simulink model "LAB4"  (R2023b)
settings: Solver=FixedStepDiscrete  StartTime=0.0  StopTime=Inf  FixedStep=0.02  RelTol=1e-3  EnableMultiTasking=on
model workspace (MAT data in the model file):
  SL_ROS_VariableLengthArrays_MaxSizes : object (value not decoded)
values from neighbouring files (symbols this model uses):
  x = x + offset    [lab4.m]    (also in occupancy_map.m; occupancy_map2.m)
  x_path = x_path(4:4:end)    [lab4.m]
  y = y + offset    [lab4.m]    (also in occupancy_map.m; occupancy_map2.m)
  y_path = y_path(4:4:end)    [lab4.m]
undefined symbols (not defined in the file or in its folder): angdiff, Angular, Linear
libraries: simulink x5, robotlib x4, robotcorelib x1, simulink_extras x1
(part 2 of 2)

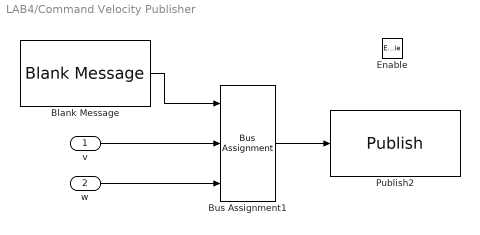
== system LAB4/Command Velocity Publisher ==
  v : Inport
  w : Inport  Port=2
  Enable : EnablePort
  Blank Message : robotlib/Blank Message  messageClass=Message  entityType=geometry_msgs/Twist  messageType=geometry_msgs/Twist  SampleTime=inf  legacyBusStruct=off
  Bus Assignment1 : BusAssignment  DialogController=Simulink.DDGSource_BusAssignment  AssignedSignals=Linear.X,Angular.Z
  Publish2 : robotlib/Publish  topicSource=Select from ROS network  topic=/cmd_vel  messageType=geometry_msgs/Twist  legacyBusStruct=off  messageQueueLength=105
  wires:
  Bus Assignment1/1 -> Publish2/1
  Blank Message/1 -> Bus Assignment1/1
  v/1 -> Bus Assignment1/2
  w/1 -> Bus Assignment1/3

== system LAB4/More Info ==

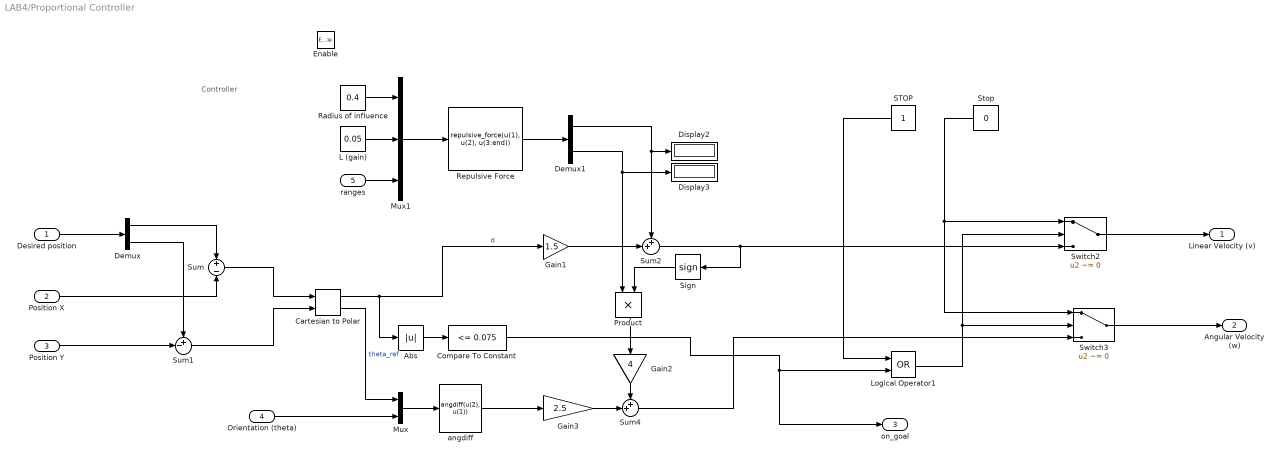
== system LAB4/Proportional Controller ==
  note: Controller
  Desired position : Inport
  Position X : Inport  Port=2
  Position Y : Inport  Port=3
  Orientation (theta) : Inport  Port=4
  ranges : Inport  Port=5
  Enable : EnablePort
  Abs : Abs  SaturateOnIntegerOverflow=off
  Cartesian to Polar : simulink_extras/Transformations/Cartesian to Polar
  Compare To Constant : simulink/Logic and Bit Operations/Compare To Constant  relop=<=  const=0.075  OutDataTypeStr=boolean
  Demux : Demux  Outputs=2
  Demux1 : Demux  Outputs=2
  Display2 : Display
  Display3 : Display
  Gain1 : Gain  Gain=1.5
  Gain2 : Gain  Gain=4
  Gain3 : Gain  Gain=2.5
  L (gain) : Constant  Value=0.05
  Logical Operator1 : Logic  Operator=OR  AllPortsSameDT=off  OutDataTypeStr=boolean
  Mux : Mux  Inputs=2
  Mux1 : Mux  Inputs=3
  Product : Product
  Radius of influence : Constant  Value=0.4
  Repulsive Force : MATLABFcn  MATLABFcn=repulsive_force(u(1), u(2), u(3:end))
      mask Display: image('baggegangsta.png');
  "STOP " : Constant
  Sign : Signum
  Stop : Constant  Value=0
  Sum : Sum  Inputs=+-
  Sum1 : Sum  Inputs=+-|
  Sum2 : Sum  Inputs=++|
  Sum4 : Sum  Inputs=++|
  Switch2 : Switch  Criteria=u2 ~= 0  SaturateOnIntegerOverflow=off  InputSameDT=off
  Switch3 : Switch  Criteria=u2 ~= 0  SaturateOnIntegerOverflow=off  InputSameDT=off
  angdiff : MATLABFcn  MATLABFcn=angdiff(u(2), u(1))
      mask Display: image('1000yardstare.PNG');
  Linear Velocity (v) : Outport  VectorParamsAs1DForOutWhenUnconnected=off
  Angular Velocity (w) : Outport  Port=2  VectorParamsAs1DForOutWhenUnconnected=off
  on_goal : Outport  Port=3
  wires:
  Stop/1 -> Switch2/1, Switch3/1
  "STOP "/1 -> Logical Operator1/1
  Switch2/1 -> Linear Velocity (v)/1
  Switch3/1 -> Angular Velocity (w)/1
  Sum2/1 -> Sign/1, Switch2/3
  Desired position/1 -> Demux/1
  Position X/1 -> Sum/2
  Position Y/1 -> Sum1/2
  Orientation (theta)/1 -> Mux/2
  Demux/1 -> Sum/1
  Demux/2 -> Sum1/1
  Sum1/1 -> Cartesian to Polar/2
  Sum/1 -> Cartesian to Polar/1
  Cartesian to Polar/2 -> Mux/1  "theta_ref"
  Mux/1 -> angdiff/1
  Cartesian to Polar/1 -> Gain1/1, Abs/1  "d"
  Gain1/1 -> Sum2/2
  angdiff/1 -> Gain3/1
  ranges/1 -> Mux1/3
  L (gain)/1 -> Mux1/2
  Radius of influence/1 -> Mux1/1
  Mux1/1 -> Repulsive Force/1
  Repulsive Force/1 -> Demux1/1
  Demux1/1 -> Sum2/1, Display2/1
  Gain3/1 -> Sum4/2
  Demux1/2 -> Product/1, Display3/1
  Product/1 -> Gain2/1
  Sign/1 -> Product/2
  Gain2/1 -> Sum4/1
  Sum4/1 -> Switch3/3
  Abs/1 -> Compare To Constant/1
  Compare To Constant/1 -> on_goal/1, Logical Operator1/2
  Logical Operator1/1 -> Switch2/2, Switch3/2

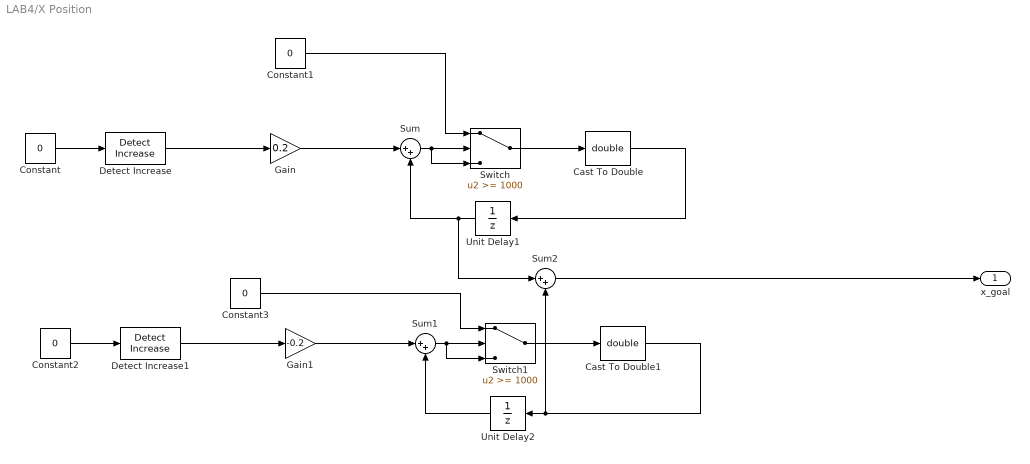
== system LAB4/X Position ==
  Cast To Double : DataTypeConversion  OutDataTypeStr=double  SaturateOnIntegerOverflow=off  RndMeth=Floor
  Cast To Double1 : DataTypeConversion  OutDataTypeStr=double  SaturateOnIntegerOverflow=off  RndMeth=Floor
  Constant{,1..3} (4 alike) : Constant  Value=0
  Detect Increase : simulink/Logic and Bit Operations/Detect Increase  vinit=0.0  OutDataTypeStr=boolean
  Detect Increase1 : simulink/Logic and Bit Operations/Detect Increase  vinit=0.0  OutDataTypeStr=boolean
  Gain : Gain  Gain=0.2
  Gain1 : Gain  Gain=-0.2
  Sum : Sum  Inputs=|++
  Sum1 : Sum  Inputs=|++
  Sum2 : Sum  Inputs=|++
  Switch : Switch  Threshold=1000  SaturateOnIntegerOverflow=off  InputSameDT=off
  Switch1 : Switch  Threshold=1000  SaturateOnIntegerOverflow=off  InputSameDT=off
  Unit Delay1 : UnitDelay  SampleTime=-1  HasFrameUpgradeWarning=on
  Unit Delay2 : UnitDelay  SampleTime=-1  HasFrameUpgradeWarning=on
  x_goal : Outport
  wires:
  Constant3/1 -> Switch1/1
  Gain1/1 -> Sum1/1
  Sum/1 -> Switch/3, Switch/2
  Gain/1 -> Sum/1
  Constant1/1 -> Switch/1
  Switch1/1 -> Cast To Double1/1
  Cast To Double/1 -> Unit Delay1/1
  Detect Increase/1 -> Gain/1
  Sum1/1 -> Switch1/3, Switch1/2
  Switch/1 -> Cast To Double/1
  Detect Increase1/1 -> Gain1/1
  Cast To Double1/1 -> Sum2/2, Unit Delay2/1
  Unit Delay2/1 -> Sum1/2
  Constant2/1 -> Detect Increase1/1
  Unit Delay1/1 -> Sum2/1, Sum/2
  Constant/1 -> Detect Increase/1
  Sum2/1 -> x_goal/1

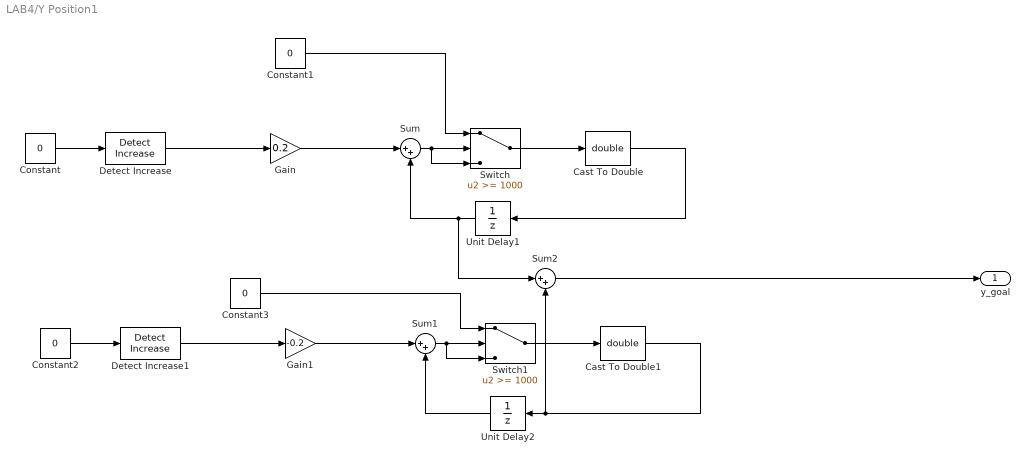
== system LAB4/Y Position1 ==
  Cast To Double : DataTypeConversion  OutDataTypeStr=double  SaturateOnIntegerOverflow=off  RndMeth=Floor
  Cast To Double1 : DataTypeConversion  OutDataTypeStr=double  SaturateOnIntegerOverflow=off  RndMeth=Floor
  Constant{,1..3} (4 alike) : Constant  Value=0
  Detect Increase : simulink/Logic and Bit Operations/Detect Increase  vinit=0.0  OutDataTypeStr=boolean
  Detect Increase1 : simulink/Logic and Bit Operations/Detect Increase  vinit=0.0  OutDataTypeStr=boolean
  Gain : Gain  Gain=0.2
  Gain1 : Gain  Gain=-0.2
  Sum : Sum  Inputs=|++
  Sum1 : Sum  Inputs=|++
  Sum2 : Sum  Inputs=|++
  Switch : Switch  Threshold=1000  SaturateOnIntegerOverflow=off  InputSameDT=off
  Switch1 : Switch  Threshold=1000  SaturateOnIntegerOverflow=off  InputSameDT=off
  Unit Delay1 : UnitDelay  SampleTime=-1  HasFrameUpgradeWarning=on
  Unit Delay2 : UnitDelay  SampleTime=-1  HasFrameUpgradeWarning=on
  y_goal : Outport
  wires:
  Constant3/1 -> Switch1/1
  Gain1/1 -> Sum1/1
  Sum/1 -> Switch/3, Switch/2
  Gain/1 -> Sum/1
  Constant1/1 -> Switch/1
  Switch1/1 -> Cast To Double1/1
  Cast To Double/1 -> Unit Delay1/1
  Detect Increase/1 -> Gain/1
  Sum1/1 -> Switch1/3, Switch1/2
  Switch/1 -> Cast To Double/1
  Detect Increase1/1 -> Gain1/1
  Cast To Double1/1 -> Sum2/2, Unit Delay2/1
  Unit Delay2/1 -> Sum1/2
  Constant2/1 -> Detect Increase1/1
  Unit Delay1/1 -> Sum2/1, Sum/2
  Constant/1 -> Detect Increase/1
  Sum2/1 -> y_goal/1

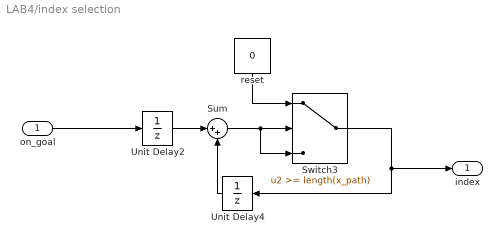
== system LAB4/index selection ==
  on_goal : Inport
  Sum : Sum  Inputs=|++
  Switch3 : Switch  Threshold=length(x_path)  SaturateOnIntegerOverflow=off  InputSameDT=off
  Unit Delay2 : UnitDelay  SampleTime=-1  HasFrameUpgradeWarning=on
  Unit Delay4 : UnitDelay  SampleTime=-1  HasFrameUpgradeWarning=on
  reset : Constant  Value=0  VectorParams1D=off
  index : Outport
  wires:
  Sum/1 -> Switch3/3, Switch3/2
  Unit Delay4/1 -> Sum/2
  reset/1 -> Switch3/1
  Switch3/1 -> index/1, Unit Delay4/1
  Unit Delay2/1 -> Sum/1
  on_goal/1 -> Unit Delay2/1
